simulink model "gm_simulink_implementation"  (R2019b)
settings: Solver=FixedStepDiscrete  StartTime=0.0  StopTime=timetorun  RelTol=1e-3
undefined symbols (not defined in the file or in its folder): sample_rate
libraries: simulink x3, hdlmdlgenlib x2, dspsrcs4 x1
settings Model: Creator=ian  LastModifiedBy=ian
settings DataIOCC: LimitDataPoints=on  SaveOutput=off  SaveTime=off
settings OptimizationCC: BlockReduction=off  ConditionallyExecuteInputs=off  DefaultParameterBehavior=Inlined  LifeSpan=inf
settings DebuggingCC: SignalRangeChecking=warning  AlgebraicLoopMsg=error  InheritedTsInSrcMsg=none  SingleTaskRateTransMsg=error  AllowSymbolicDim=off  StrictBusMsg=ErrorOnBusTreatedAsVector  SFUnexpectedBacktrackingDiag=warning  SFNoUnconditionalDefaultTransitionDiag=warning  SFExecutionAtInitializationDiag=none  ArithmeticOperatorsInVariantConditions=warning
settings HardwareCC: ProdBitPerPointer=32  ProdBitPerSizeT=32  ProdBitPerPtrDiffT=32  ProdLargestAtomicFloat=None  ProdIntDivRoundTo=Undefined  ProdEndianess=Unspecified  ProdWordSize=32  ProdHWDeviceType=ASIC/FPGA->ASIC/FPGA  TargetBitPerPointer=64  TargetBitPerSizeT=64  TargetBitPerPtrDiffT=64  TargetLongLongMode=on  TargetIntDivRoundTo=Zero  TargetEndianess=LittleEndian  TargetWordSize=64  TargetHWDeviceType=Custom Processor->MATLAB Host Computer  ProdEqTarget=off
settings SFSimCC: SimUseLocalCustomCode=off  CustomCodeUndefinedFunction=UseInterfaceOnly
settings RTWCC: RTWUseLocalCustomCode=off
settings CodeAppCC: StateflowObjectComments=on
settings GRTTargetCC: TargetLangStandard=C89/C90 (ANSI)  GeneratePreprocessorConditionals=Disable all
settings ConfigComp: CovScope=ReferencedModels  CovMetricSettings=dw  CovHtmlReporting=on  CovSaveCumulativeToWorkspaceVar=on  CovSaveSingleToWorkspaceVar=on  CovExternalEMLEnable=off  CovSFcnEnable=off

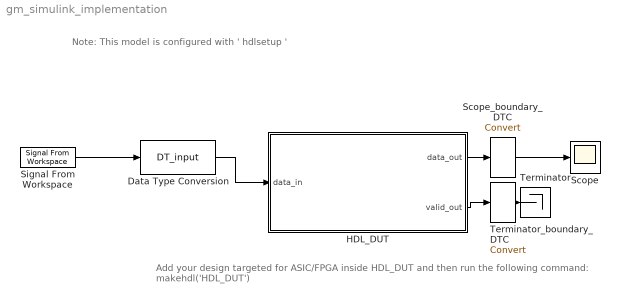
== system gm_simulink_implementation ==
  note: Add your design targeted for ASIC/FPGA inside HDL_DUT and then run the following command:
      | makehdl('HDL_DUT')
  note: Note: This model is configured with ' hdlsetup '
  Data Type Conversion : DataTypeConversion  OutDataTypeStr=DT_input
  HDL_DUT : Subsystem
  Scope : Scope
  Scope_boundary_DTC : DataTypeConversion  SaturateOnIntegerOverflow=on  RndMeth=Zero
  Signal From Workspace : dspsrcs4/Signal From Workspace  X=v_in  Ts=sample_rate  nsamps=dsp_slices  OutputAfterFinalValue=Setting to zero  ignoreOrWarnInputAndFrameLengths=off  OutputFrames=off
  Terminator : Terminator
  Terminator_boundary_DTC : DataTypeConversion  SaturateOnIntegerOverflow=on  RndMeth=Zero
  wires:
  Terminator_boundary_DTC/1 -> Terminator/1
  HDL_DUT/2(valid_out) -> Terminator_boundary_DTC/1
  Scope_boundary_DTC/1 -> Scope/1
  HDL_DUT/1(data_out) -> Scope_boundary_DTC/1
  Data Type Conversion/1 -> HDL_DUT/1(data_in)
  Signal From Workspace/1 -> Data Type Conversion/1

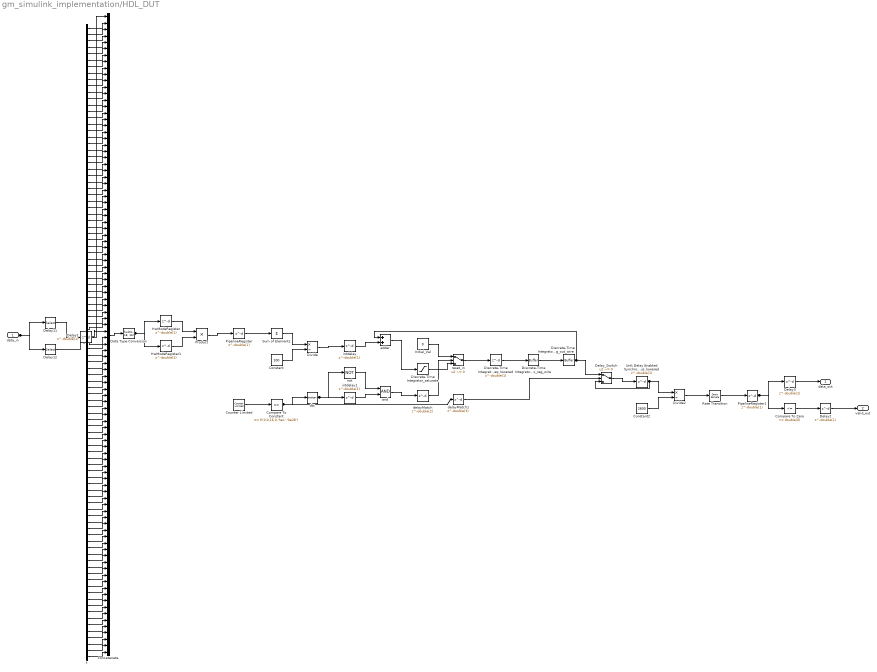
== system gm_simulink_implementation/HDL_DUT ==
  data_in : Inport  OutDataTypeStr=fixdt(1, 12, 10)  PortDimensions=[100 1]  SampleTime=3.84615384615385e-08
  Compare To Constant : simulink/Logic and Bit Operations/Compare To Constant  relop===  const=fi(0,0,16,0,'hex','0a28')  OutDataTypeStr=boolean
  Compare To Zero : simulink/Logic and Bit Operations/Compare To Constant  relop=<=  const=double(0)  OutDataTypeStr=boolean
  Constant : Constant  Value=100  OutDataTypeStr=uint16  SampleTime=-1
  Constant2 : Constant  Value=2600  OutDataTypeStr=uint16  SampleTime=-1
  Counter Limited : simulink/Sources/Counter Limited  uplimit=double(2600)  tsamp=3.84615384615385e-08
  Data Type Conversion : DataTypeConversion  OutDataTypeStr=fixdt(1, 18, 16)  RndMeth=Nearest  SampleTime=3.84615384615385e-08
  Delay1 : Delay  DelayLength=double(1)  InitialCondition=0  SampleTime=3.84615384615385e-08
  Delay11 : Selector  IndexMode=Zero-based  SampleTime=3.84615384615385e-08  IndexOptions=Index vector (dialog)  Indices=99  OutputSizes=1
  Delay12 : Selector  IndexMode=Zero-based  SampleTime=3.84615384615385e-08  IndexOptions=Index vector (dialog)  Indices=uint32([0 1 2 3 4 5 6 7 8 9 10 11 12 13 14 15 16 17 18 19 20 21 22 23 24 25 26 27 28 29 30 31 32 33 34 35 36 37 38 39 40 41 42 43 44 45 46 47 48 49 50 51 52 53 54 55 56 57 58 59 60 61 62 63 64 65 66 67 68 69 70 71 72 73 74 75 76 77 78 79 80 81 82 83 84 85 86 87 88 89 90 91 92 93 94 95 96 97 98])  OutputSizes=1
  Delay2 : Delay  DelayLength=double(1)  InitialCondition=0  SampleTime=0.0001
  Delay3 : Delay  DelayLength=double(1)  InitialCondition=0  SampleTime=0.0001
  Delay_Switch : Switch  Criteria=u2 ~= 0  Threshold=double(0)  OutDataTypeStr=fixdt(1, 43, 32)  SampleTime=3.84615384615385e-08
  Discrete-Time Integrator_reg_lowered : Delay  DelayLength=double(1)  InitialCondition=0  SampleTime=3.84615384615385e-08
  Discrete-Time Integrator_saturate : Saturate  UpperLimit=fi(0,1,43,32,'hex','3e800000000')  LowerLimit=fi(0,1,43,32,'hex','00000000000')  SampleTime=3.84615384615385e-08  OutDataTypeStr=fixdt(1, 43, 32)
  Discrete-Time Integrator_x_reg_out_wire : hdlmdlgenlib/Buffer
      settings: SourceProductName=Simulink  SourceProductBaseCode=SL
  Discrete-Time Integrator_x_reg_wire : hdlmdlgenlib/Buffer
      settings: SourceProductName=Simulink  SourceProductBaseCode=SL
  Divide : Product  Inputs=*/  OutDataTypeStr=fixdt(1, 43, 32)  SampleTime=3.84615384615385e-08  SaturateOnIntegerOverflow=on  RndMeth=Zero
  Divide2 : Product  Inputs=*/  OutDataTypeStr=fixdt(1, 43, 32)  RndMeth=Simplest  SampleTime=3.84615384615385e-08  SaturateOnIntegerOverflow=on
  HwModeRegister : Delay  DelayLength=double(1)  InitialCondition=0  SampleTime=3.84615384615385e-08
  HwModeRegister1 : Delay  DelayLength=double(1)  InitialCondition=0  SampleTime=3.84615384615385e-08
  Initial_Val : Constant  Value=0  OutDataTypeStr=fixdt(1, 43, 32)  SampleTime=-1
  PipelineRegister : Delay  DelayLength=double(1)  InitialCondition=0  SampleTime=3.84615384615385e-08
  PipelineRegister1 : Delay  DelayLength=double(1)  InitialCondition=0  SampleTime=0.0001
  Product : Product  Inputs=**  OutDataTypeStr=fixdt(1, 36, 32)  SampleTime=3.84615384615385e-08
  Rate Transition : DownSample  N=double(2600)  phase=double(3)  RateOptions=Allow multirate processing
  Sum of Elements : Sum  Inputs=+  AccumDataTypeStr=fixdt(1, 43, 32)  OutDataTypeStr=fixdt(1, 43, 32)  SampleTime=3.84615384615385e-08
  Unit Delay Enabled Synchronous_lowered : Delay  DelayLength=double(1)  InitialCondition=0  SampleTime=3.84615384615385e-08
  adder : Sum  AccumDataTypeStr=fixdt(1, 43, 32)  OutDataTypeStr=fixdt(1, 43, 32)  SampleTime=3.84615384615385e-08
  and : Logic  AllPortsSameDT=off  OutDataTypeStr=boolean  SampleTime=3.84615384615385e-08
  concatenate : Concatenate  NumInputs=100
  delayMatch : Delay  DelayLength=double(2)  InitialCondition=0  SampleTime=3.84615384615385e-08
  delayMatch1 : Delay  DelayLength=double(3)  InitialCondition=0  SampleTime=3.84615384615385e-08
  dtc : DataTypeConversion  OutDataTypeStr=boolean  SampleTime=3.84615384615385e-08
  intdelay : Delay  DelayLength=double(1)  InitialCondition=0  SampleTime=3.84615384615385e-08
  intdelay1 : Delay  DelayLength=double(1)  InitialCondition=0  SampleTime=3.84615384615385e-08
  not : Logic  Operator=NOT  Inputs=1  AllPortsSameDT=off  OutDataTypeStr=boolean  SampleTime=3.84615384615385e-08
  reset_in : Switch  Criteria=u2 ~= 0  Threshold=double(0)  OutDataTypeStr=fixdt(1, 43, 32)  SampleTime=3.84615384615385e-08
  t : Demux  Outputs=99
  data_out : Outport  VectorParamsAs1DForOutWhenUnconnected=off
  valid_out : Outport  Port=2  VectorParamsAs1DForOutWhenUnconnected=off
  wires:
  data_in/1 -> Delay11/1, Delay12/1
  Compare To Zero/1 -> Delay2/1
  Counter Limited/1 -> Compare To Constant/1
  Delay2/1 -> valid_out/1
  Delay3/1 -> data_out/1
  Divide/1 -> intdelay/1
  PipelineRegister1/1 -> Compare To Zero/1, Delay3/1
  Delay11/1 -> Delay1/1
  Delay1/1 -> concatenate/1
  intdelay/1 -> adder/2
  dtc/1 -> intdelay1/1, not/1
  intdelay1/1 -> and/2
  Initial_Val/1 -> reset_in/1
  delayMatch/1 -> reset_in/2
  not/1 -> and/1
  delayMatch1/1 -> Delay_Switch/2
  Delay12/1 -> t/1
  t/1 -> concatenate/2
  t/2 -> concatenate/3
  t/3 -> concatenate/4
  t/4 -> concatenate/5
  t/5 -> concatenate/6
  t/6 -> concatenate/7
  t/7 -> concatenate/8
  t/8 -> concatenate/9
  t/9 -> concatenate/10
  t/10 -> concatenate/11
  t/11 -> concatenate/12
  t/12 -> concatenate/13
  t/13 -> concatenate/14
  t/14 -> concatenate/15
  t/15 -> concatenate/16
  t/16 -> concatenate/17
  t/17 -> concatenate/18
  t/18 -> concatenate/19
  t/19 -> concatenate/20
  t/20 -> concatenate/21
  t/21 -> concatenate/22
  t/22 -> concatenate/23
  t/23 -> concatenate/24
  t/24 -> concatenate/25
  t/25 -> concatenate/26
  t/26 -> concatenate/27
  t/27 -> concatenate/28
  t/28 -> concatenate/29
  t/29 -> concatenate/30
  t/30 -> concatenate/31
  t/31 -> concatenate/32
  t/32 -> concatenate/33
  t/33 -> concatenate/34
  t/34 -> concatenate/35
  t/35 -> concatenate/36
  t/36 -> concatenate/37
  t/37 -> concatenate/38
  t/38 -> concatenate/39
  t/39 -> concatenate/40
  t/40 -> concatenate/41
  t/41 -> concatenate/42
  t/42 -> concatenate/43
  t/43 -> concatenate/44
  t/44 -> concatenate/45
  t/45 -> concatenate/46
  t/46 -> concatenate/47
  t/47 -> concatenate/48
  t/48 -> concatenate/49
  t/49 -> concatenate/50
  t/50 -> concatenate/51
  t/51 -> concatenate/52
  t/52 -> concatenate/53
  t/53 -> concatenate/54
  t/54 -> concatenate/55
  t/55 -> concatenate/56
  t/56 -> concatenate/57
  t/57 -> concatenate/58
  t/58 -> concatenate/59
  t/59 -> concatenate/60
  t/60 -> concatenate/61
  t/61 -> concatenate/62
  t/62 -> concatenate/63
  t/63 -> concatenate/64
  t/64 -> concatenate/65
  t/65 -> concatenate/66
  t/66 -> concatenate/67
  t/67 -> concatenate/68
  t/68 -> concatenate/69
  t/69 -> concatenate/70
  t/70 -> concatenate/71
  t/71 -> concatenate/72
  t/72 -> concatenate/73
  t/73 -> concatenate/74
  t/74 -> concatenate/75
  t/75 -> concatenate/76
  t/76 -> concatenate/77
  t/77 -> concatenate/78
  t/78 -> concatenate/79
  t/79 -> concatenate/80
  t/80 -> concatenate/81
  t/81 -> concatenate/82
  t/82 -> concatenate/83
  t/83 -> concatenate/84
  t/84 -> concatenate/85
  t/85 -> concatenate/86
  t/86 -> concatenate/87
  t/87 -> concatenate/88
  t/88 -> concatenate/89
  t/89 -> concatenate/90
  t/90 -> concatenate/91
  t/91 -> concatenate/92
  t/92 -> concatenate/93
  t/93 -> concatenate/94
  t/94 -> concatenate/95
  t/95 -> concatenate/96
  t/96 -> concatenate/97
  t/97 -> concatenate/98
  t/98 -> concatenate/99
  t/99 -> concatenate/100
  concatenate/1 -> Data Type Conversion/1
  Data Type Conversion/1 -> HwModeRegister/1, HwModeRegister1/1
  PipelineRegister/1 -> Sum of Elements/1
  Sum of Elements/1 -> Divide/1
  Constant/1 -> Divide/2
  Constant2/1 -> Divide2/2
  and/1 -> delayMatch/1
  Compare To Constant/1 -> delayMatch1/1, dtc/1
  Divide2/1 -> Rate Transition/1
  adder/1 -> Discrete-Time Integrator_saturate/1
  Discrete-Time Integrator_saturate/1 -> reset_in/3
  reset_in/1 -> Discrete-Time Integrator_reg_lowered/1
  Discrete-Time Integrator_reg_lowered/1 -> Discrete-Time Integrator_x_reg_wire/1
  Discrete-Time Integrator_x_reg_wire/1 -> Discrete-Time Integrator_x_reg_out_wire/1
  Discrete-Time Integrator_x_reg_out_wire/1 -> adder/1, Delay_Switch/1
  Delay_Switch/1 -> Unit Delay Enabled Synchronous_lowered/1
  Unit Delay Enabled Synchronous_lowered/1 -> Delay_Switch/3, Divide2/1
  Product/1 -> PipelineRegister/1
  HwModeRegister/1 -> Product/1
  HwModeRegister1/1 -> Product/2
  Rate Transition/1 -> PipelineRegister1/1
